simulink model "ex1c_Va"  (R2015a)
settings: Solver=ode45  StartTime=0.0  StopTime=100.0  RelTol=1e-3
values from neighbouring files (symbols this model uses):
  A = [-Ra/La -Kg/La ; Km/J -D/J]    [ex1c.m]
  B = [1/La 0 ; 0 -1/J]    [ex1c.m]
  C = [0 60/(2*pi) ; 1 0]    [ex1c.m]
  D = [0 0 ; 0 0]    [ex1c.m]
  TL = 5    [ex1c.m]
  Va = 10    [ex1c.m]
settings Model: Creator=martinspedro  LastModifiedBy=martinspedro

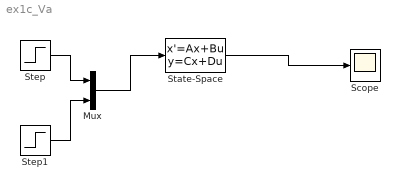
== system ex1c_Va ==
  Mux : Mux  Inputs=2
  Scope : Scope
      settings: ShowLegends=on
  State-Space : StateSpace  A=A  B=B  C=C  D=D  X0=0
  Step : Step  Time=0  After=Va  SampleTime=0
  Step1 : Step  Time=50  After=TL  SampleTime=0
  wires:
  State-Space/1 -> Scope/1
  Step/1 -> Mux/1
  Step1/1 -> Mux/2
  Mux/1 -> State-Space/1
